simulink model "Simulator_3D"  (R2018a)
settings: Solver=ode4  StartTime=0.0  StopTime=80  FixedStep=T  RelTol=1e-3
values from neighbouring files (symbols this model uses):
  A_w = 1*1.5/2    (= 0.75)    [init_Simulator.m]
  A_w2 = 1*0.27/2    (= 0.135)    [init_Simulator.m]
  epsilon_w = 0    [init_Simulator.m]
  epsilon_w2 = pi    (= 3.14159265359)    [init_Simulator.m]
  k_w = omega_w^2/g    (= 0.123862835563)    [init_Simulator.m]
  k_w2 = omega_w2^2/g    (= 0.447144836384)    [init_Simulator.m]
  Lc_0 = 7    [init_Simulator.m]
  omega_w = 2*pi/T_w    (= 1.10231321179)    [init_Simulator.m]
  omega_w2 = 2*pi/T_w2    (= 2.09439510239)    [init_Simulator.m]
  T = 1/30    (= 0.0333333333333)    [init_Simulator.m]
  w_dir = 1    [init_Simulator.m]
  w_dir2 = 1    [init_Simulator.m]
  zu_bar = X0_b(2) + Lc_0*sin(alpha_bar_0)    [init_Simulator.m]
libraries: vrlib x132
(part 2 of 6)

== system Simulator_3D/Subsystem/5 static wave points6 ==
  t : Inport
  x : Inport  Port=2
  Bias{23,25,27,29,31} (5 alike) : Bias  Bias=10
  Bias{24,26,28,30,32} (5 alike) : Bias  Bias=1
  Display : Display
  Divide : Product  Inputs=*/
  Mux{11..15} (5 alike) : Mux  Inputs=2
  Product : Product
  Round : Rounding
  Subsystem12 : Subsystem
  Subsystem13 : Subsystem
  Subsystem14 : Subsystem
  Subsystem15 : Subsystem
  Subsystem16 : Subsystem
  Sum{,1..4} (5 alike) : Sum  Inputs=|++
  Viewpoint {12..16} (5 alike) : vrlib/VR Signal Expander  outwidth=3  outidx=[1 2]
      settings: SourceProductName=Simulink 3D Animation  SourceProductBaseCode=VR
  reference : Constant  Value=5+3
  window width : Constant  Value=10
  Out1 : Outport
  Out2 : Outport  Port=2
  Out3 : Outport  Port=3
  Out4 : Outport  Port=4
  Out5 : Outport  Port=5
  Out6 : Outport  Port=6
  Out7 : Outport  Port=7
  Out8 : Outport  Port=8
  Out9 : Outport  Port=9
  Out10 : Outport  Port=10
  wires:
  Sum2/1 -> Subsystem15/2(x), Mux14/1
  Sum1/1 -> Subsystem13/2(x), Mux12/1
  Sum3/1 -> Subsystem14/2(x), Mux13/1
  Subsystem14/2(theta) -> Out6/1
  Subsystem13/2(theta) -> Out4/1
  Bias27/1 -> Mux13/2
  Mux13/1 -> Viewpoint 14/1
  Subsystem13/1(zeta) -> Bias25/1
  Subsystem16/2(theta) -> Out10/1
  Mux12/1 -> Viewpoint 13/1
  Bias23/1 -> Mux11/2
  Mux11/1 -> Viewpoint 12/1
  Subsystem14/1(zeta) -> Bias27/1
  Bias25/1 -> Mux12/2
  Subsystem15/2(theta) -> Out8/1
  Mux15/1 -> Viewpoint 16/1
  Bias31/1 -> Mux15/2
  Viewpoint 16/1 -> Out9/1
  Sum4/1 -> Subsystem16/2(x), Mux15/1
  Subsystem12/2(theta) -> Out2/1
  Subsystem16/1(zeta) -> Bias31/1
  Bias29/1 -> Mux14/2
  Sum/1 -> Subsystem12/2(x), Mux11/1
  Mux14/1 -> Viewpoint 15/1
  Viewpoint 12/1 -> Display/1, Out1/1
  Subsystem12/1(zeta) -> Bias23/1
  Viewpoint 15/1 -> Out7/1
  Subsystem15/1(zeta) -> Bias29/1
  t/1 -> Subsystem15/1(t), Subsystem16/1(t), Subsystem14/1(t), Subsystem13/1(t), Subsystem12/1(t)
  Round/1 -> Product/2
  Divide/1 -> Round/1
  x/1 -> Divide/1
  window width/1 -> Divide/2, Product/1
  Bias24/1 -> Bias26/1, Sum/1
  reference/1 -> Bias24/1
  Product/1 -> Sum4/2, Sum2/2, Sum3/2, Sum1/2, Sum/2
  Bias26/1 -> Bias28/1, Sum1/1
  Bias32/1 -> Sum4/1
  Bias30/1 -> Bias32/1, Sum2/1
  Bias28/1 -> Bias30/1, Sum3/1
  Viewpoint 13/1 -> Out3/1
  Viewpoint 14/1 -> Out5/1

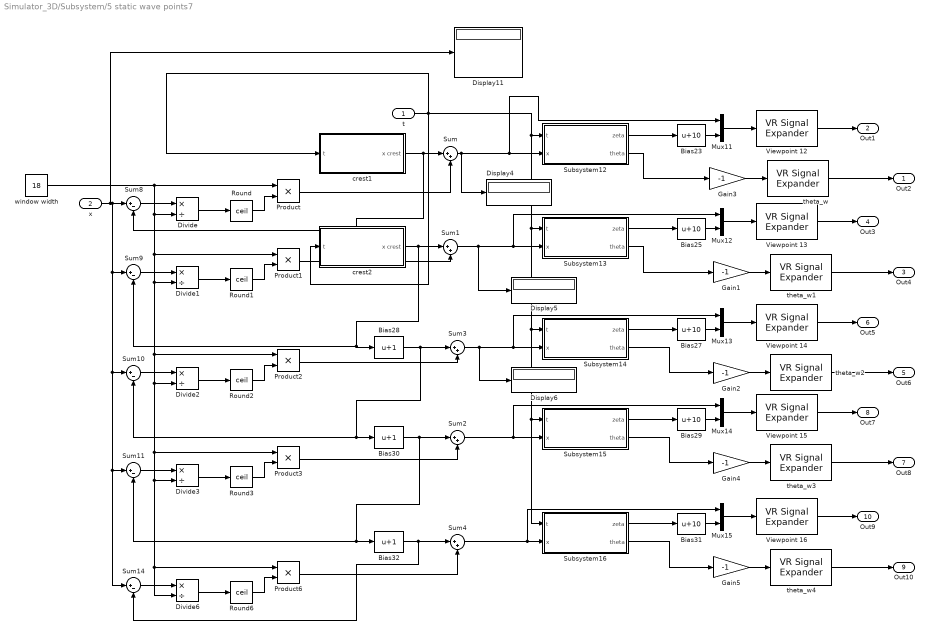
== system Simulator_3D/Subsystem/5 static wave points7 ==
  t : Inport
  x : Inport  Port=2
  Bias{23,25,27,29,31} (5 alike) : Bias  Bias=10
  Bias28 : Bias  Bias=1
  Bias30 : Bias  Bias=1
  Bias32 : Bias  Bias=1
  Display{4..6,11} (4 alike) : Display
  Divide{,1..3,6} (5 alike) : Product  Inputs=*/
  Gain{1..5} (5 alike) : Gain  Gain=-1
  Mux{11..15} (5 alike) : Mux  Inputs=2
  Product{,1..3,6} (5 alike) : Product
  Round{,1..3,6} (5 alike) : Rounding  Operator=ceil
  Subsystem12 : Subsystem
  Subsystem13 : Subsystem
  Subsystem14 : Subsystem
  Subsystem15 : Subsystem
  Subsystem16 : Subsystem
  Sum{,1..4} (5 alike) : Sum  Inputs=|++
  Sum{8..11,14} (5 alike) : Sum  Inputs=|+-
  Viewpoint {12..16} (5 alike) : vrlib/VR Signal Expander  outwidth=3  outidx=[1 2]
      settings: SourceProductName=Simulink 3D Animation  SourceProductBaseCode=VR
  crest1 : Subsystem
  crest2 : Subsystem
  theta_w{,1..4} (5 alike) : vrlib/VR Signal Expander  outwidth=4  outidx=[4]
      settings: SourceProductName=Simulink 3D Animation  SourceProductBaseCode=VR
  window width : Constant  Value=18
  Out2 : Outport
  Out1 : Outport  Port=2
  Out4 : Outport  Port=3
  Out3 : Outport  Port=4
  Out6 : Outport  Port=5
  Out5 : Outport  Port=6
  Out8 : Outport  Port=7
  Out7 : Outport  Port=8
  Out10 : Outport  Port=9
  Out9 : Outport  Port=10
  wires:
  x/1 -> Sum8/1, Sum9/1, Sum10/1, Sum11/1, Sum14/1, Display11/1
  window width/1 -> Product/1, Divide/2, Product1/1, Divide1/2, Divide2/2, Divide3/2, Product6/1, Divide6/2, Product3/1, Product2/1
  Round6/1 -> Product6/2
  Divide6/1 -> Round6/1
  Sum14/1 -> Divide6/1
  Product6/1 -> Sum4/2
  Bias32/1 -> Sum4/1, Sum14/2
  Product3/1 -> Sum2/2
  Sum11/1 -> Divide3/1
  Divide3/1 -> Round3/1
  Round3/1 -> Product3/2
  Bias30/1 -> Bias32/1, Sum11/2, Sum2/1
  Bias28/1 -> Sum3/1, Sum10/2, Bias30/1
  Round2/1 -> Product2/2
  Divide2/1 -> Round2/1
  Sum10/1 -> Divide2/1
  Product2/1 -> Sum3/2
  Product1/1 -> Sum1/2
  Sum9/1 -> Divide1/1
  Divide1/1 -> Round1/1
  Round1/1 -> Product1/2
  crest2/1(x crest) -> Bias28/1, Sum9/2, Sum1/1
  crest1/1(x crest) -> Sum/1, Sum8/2
  t/1 -> crest2/1(t), crest1/1(t), Subsystem15/1(t), Subsystem16/1(t), Subsystem14/1(t), Subsystem13/1(t), Subsystem12/1(t)
  Round/1 -> Product/2
  Divide/1 -> Round/1
  Sum8/1 -> Divide/1
  Subsystem13/2(theta) -> Gain1/1
  Gain2/1 -> theta_w2/1
  Gain4/1 -> theta_w3/1
  theta_w1/1 -> Out4/1
  Subsystem16/2(theta) -> Gain5/1
  Viewpoint 15/1 -> Out7/1
  Sum2/1 -> Subsystem15/2(x), Mux14/1
  Sum1/1 -> Subsystem13/2(x), Mux12/1, Display5/1
  Sum4/1 -> Mux15/1, Subsystem16/2(x)
  Subsystem15/2(theta) -> Gain4/1
  Bias27/1 -> Mux13/2
  Bias25/1 -> Mux12/2
  Mux13/1 -> Viewpoint 14/1
  Subsystem13/1(zeta) -> Bias25/1
  Viewpoint 14/1 -> Out5/1
  Viewpoint 16/1 -> Out9/1
  Bias23/1 -> Mux11/2
  Mux15/1 -> Viewpoint 16/1
  Subsystem14/1(zeta) -> Bias27/1
  Bias31/1 -> Mux15/2
  Subsystem14/2(theta) -> Gain2/1
  Mux14/1 -> Viewpoint 15/1
  Subsystem16/1(zeta) -> Bias31/1
  Subsystem15/1(zeta) -> Bias29/1
  Sum/1 -> Mux11/1, Subsystem12/2(x), Display4/1
  Viewpoint 13/1 -> Out3/1
  Subsystem12/1(zeta) -> Bias23/1
  Gain5/1 -> theta_w4/1
  theta_w3/1 -> Out8/1
  Mux11/1 -> Viewpoint 12/1
  Subsystem12/2(theta) -> Gain3/1
  Bias29/1 -> Mux14/2
  theta_w2/1 -> Out6/1
  Gain1/1 -> theta_w1/1
  Viewpoint 12/1 -> Out1/1
  theta_w4/1 -> Out10/1
  Sum3/1 -> Subsystem14/2(x), Mux13/1, Display6/1
  theta_w/1 -> Out2/1
  Mux12/1 -> Viewpoint 13/1
  Gain3/1 -> theta_w/1
  Product/1 -> Sum/2

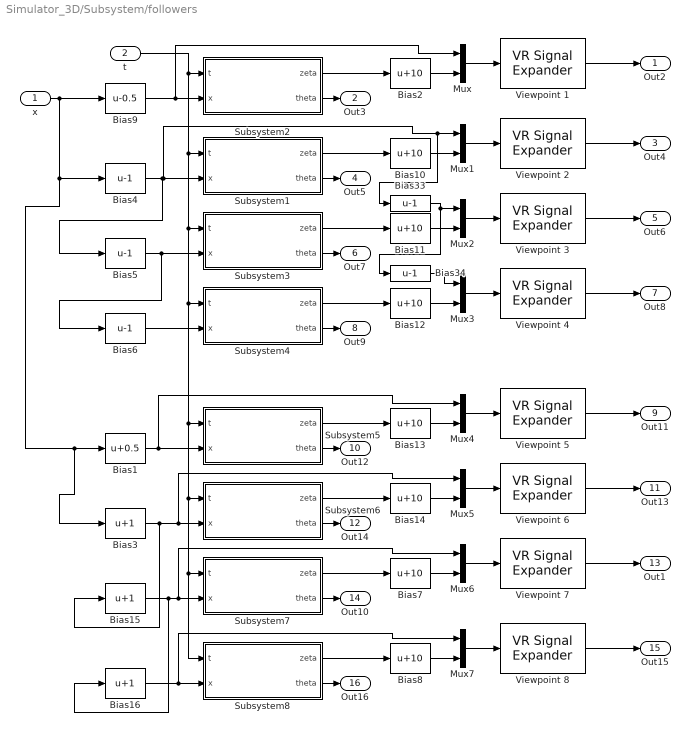
== system Simulator_3D/Subsystem/followers ==
  x : Inport
  t : Inport  Port=2
  Bias1 : Bias  Bias=0.5
  Bias{2,7..8,10..14} (8 alike) : Bias  Bias=10
  Bias15 : Bias  Bias=1
  Bias16 : Bias  Bias=1
  Bias3 : Bias  Bias=1
  Bias{4..6,33..34} (5 alike) : Bias  Bias=-1
  Bias9 : Bias  Bias=-0.5
  Mux{,1..7} (8 alike) : Mux  Inputs=2
  Subsystem1 : Subsystem
  Subsystem2 : Subsystem
  Subsystem3 : Subsystem
  Subsystem4 : Subsystem
  Subsystem5 : Subsystem
  Subsystem6 : Subsystem
  Subsystem7 : Subsystem
  Subsystem8 : Subsystem
  Viewpoint {1..8} (8 alike) : vrlib/VR Signal Expander  outwidth=3  outidx=[1 2]
      settings: SourceProductName=Simulink 3D Animation  SourceProductBaseCode=VR
  Out2 : Outport
  Out3 : Outport  Port=2
  Out4 : Outport  Port=3
  Out5 : Outport  Port=4
  Out6 : Outport  Port=5
  Out7 : Outport  Port=6
  Out8 : Outport  Port=7
  Out9 : Outport  Port=8
  Out11 : Outport  Port=9
  Out12 : Outport  Port=10
  Out13 : Outport  Port=11
  Out14 : Outport  Port=12
  Out1 : Outport  Port=13
  Out10 : Outport  Port=14
  Out15 : Outport  Port=15
  Out16 : Outport  Port=16
  wires:
  Subsystem2/2(theta) -> Out3/1
  Bias33/1 -> Bias34/1, Mux2/1
  Subsystem6/2(theta) -> Out14/1
  Mux2/1 -> Viewpoint 3/1
  Bias4/1 -> Bias5/1, Bias33/1, Mux1/1, Subsystem1/2(x)
  Mux5/1 -> Viewpoint 6/1
  Bias11/1 -> Mux2/2
  Mux/1 -> Viewpoint 1/1
  Bias13/1 -> Mux4/2
  Subsystem2/1(zeta) -> Bias2/1
  Subsystem3/1(zeta) -> Bias11/1
  Bias10/1 -> Mux1/2
  Bias34/1 -> Mux3/1
  Mux4/1 -> Viewpoint 5/1
  Bias2/1 -> Mux/2
  Mux3/1 -> Viewpoint 4/1
  Bias14/1 -> Mux5/2
  Viewpoint 4/1 -> Out8/1
  Bias5/1 -> Bias6/1, Subsystem3/2(x)
  Viewpoint 6/1 -> Out13/1
  Subsystem6/1(zeta) -> Bias14/1
  Subsystem4/1(zeta) -> Bias12/1
  Subsystem3/2(theta) -> Out7/1
  Subsystem1/1(zeta) -> Bias10/1
  Subsystem5/1(zeta) -> Bias13/1
  Bias9/1 -> Mux/1, Subsystem2/2(x)
  Viewpoint 1/1 -> Out2/1
  Bias6/1 -> Subsystem4/2(x)
  Viewpoint 2/1 -> Out4/1
  Bias12/1 -> Mux3/2
  Mux1/1 -> Viewpoint 2/1
  Subsystem4/2(theta) -> Out9/1
  Viewpoint 3/1 -> Out6/1
  Viewpoint 5/1 -> Out11/1
  Subsystem1/2(theta) -> Out5/1
  Subsystem5/2(theta) -> Out12/1
  x/1 -> Bias3/1, Bias1/1, Bias4/1, Bias9/1
  Bias1/1 -> Mux4/1, Subsystem5/2(x)
  Subsystem7/1(zeta) -> Bias7/1
  Viewpoint 7/1 -> Out1/1
  Bias7/1 -> Mux6/2
  Mux6/1 -> Viewpoint 7/1
  Bias15/1 -> Subsystem7/2(x), Mux6/1, Bias16/1
  Subsystem7/2(theta) -> Out10/1
  Subsystem8/2(theta) -> Out16/1
  Bias3/1 -> Bias15/1, Mux5/1, Subsystem6/2(x)
  Bias16/1 -> Mux7/1, Subsystem8/2(x)
  Mux7/1 -> Viewpoint 8/1
  Bias8/1 -> Mux7/2
  Viewpoint 8/1 -> Out15/1
  Subsystem8/1(zeta) -> Bias8/1
  t/1 -> Subsystem1/1(t), Subsystem3/1(t), Subsystem4/1(t), Subsystem5/1(t), Subsystem8/1(t), Subsystem7/1(t), Subsystem6/1(t), Subsystem2/1(t)

== system Simulator_3D/Subsystem1/Subsystem1 ==
  t : Inport
  x : Inport  Port=2
  Subsystem : Subsystem
  Subsystem1 : Subsystem
  Sum2 : Sum  Inputs=++|
  zeta : Outport
  wires:
  Subsystem1/1(zeta(x,t)) -> Sum2/1
  Sum2/1 -> zeta/1
  Subsystem/1(zeta(x,t)) -> Sum2/2
  t/1 -> Subsystem1/1(t), Subsystem/1(t)
  x/1 -> Subsystem1/2(x), Subsystem/2(x)

== system Simulator_3D/Subsystem1/Subsystem10 ==
  t : Inport
  x : Inport  Port=2
  Subsystem : Subsystem
  Subsystem1 : Subsystem
  Sum2 : Sum  Inputs=++|
  zeta : Outport
  wires:
  x/1 -> Subsystem/2(x), Subsystem1/2(x)
  t/1 -> Subsystem/1(t), Subsystem1/1(t)
  Subsystem/1(zeta(x,t)) -> Sum2/2
  Sum2/1 -> zeta/1
  Subsystem1/1(zeta(x,t)) -> Sum2/1

== system Simulator_3D/Subsystem1/Subsystem11 ==
  t : Inport
  x : Inport  Port=2
  Subsystem : Subsystem
  Subsystem1 : Subsystem
  Sum2 : Sum  Inputs=++|
  zeta : Outport
  wires:
  Subsystem1/1(zeta(x,t)) -> Sum2/1
  Sum2/1 -> zeta/1
  Subsystem/1(zeta(x,t)) -> Sum2/2
  t/1 -> Subsystem1/1(t), Subsystem/1(t)
  x/1 -> Subsystem1/2(x), Subsystem/2(x)

== system Simulator_3D/Subsystem1/Subsystem12 ==
  t : Inport
  x : Inport  Port=2
  Subsystem : Subsystem
  Subsystem1 : Subsystem
  Sum2 : Sum  Inputs=++|
  zeta : Outport
  wires:
  x/1 -> Subsystem/2(x), Subsystem1/2(x)
  t/1 -> Subsystem/1(t), Subsystem1/1(t)
  Subsystem/1(zeta(x,t)) -> Sum2/2
  Sum2/1 -> zeta/1
  Subsystem1/1(zeta(x,t)) -> Sum2/1

== system Simulator_3D/Subsystem1/Subsystem13 ==
  t : Inport
  x : Inport  Port=2
  Subsystem : Subsystem
  Subsystem1 : Subsystem
  Sum2 : Sum  Inputs=++|
  zeta : Outport
  wires:
  Subsystem1/1(zeta(x,t)) -> Sum2/1
  Sum2/1 -> zeta/1
  Subsystem/1(zeta(x,t)) -> Sum2/2
  t/1 -> Subsystem1/1(t), Subsystem/1(t)
  x/1 -> Subsystem1/2(x), Subsystem/2(x)

== system Simulator_3D/Subsystem1/Subsystem14 ==
  t : Inport
  x : Inport  Port=2
  Subsystem : Subsystem
  Subsystem1 : Subsystem
  Sum2 : Sum  Inputs=++|
  zeta : Outport
  wires:
  x/1 -> Subsystem/2(x), Subsystem1/2(x)
  t/1 -> Subsystem/1(t), Subsystem1/1(t)
  Subsystem/1(zeta(x,t)) -> Sum2/2
  Sum2/1 -> zeta/1
  Subsystem1/1(zeta(x,t)) -> Sum2/1

== system Simulator_3D/Subsystem1/Subsystem15 ==
  t : Inport
  x : Inport  Port=2
  Subsystem : Subsystem
  Subsystem1 : Subsystem
  Sum2 : Sum  Inputs=++|
  zeta : Outport
  wires:
  Subsystem1/1(zeta(x,t)) -> Sum2/1
  Sum2/1 -> zeta/1
  Subsystem/1(zeta(x,t)) -> Sum2/2
  t/1 -> Subsystem1/1(t), Subsystem/1(t)
  x/1 -> Subsystem1/2(x), Subsystem/2(x)

== system Simulator_3D/Subsystem1/Subsystem16 ==
  t : Inport
  x : Inport  Port=2
  Subsystem : Subsystem
  Subsystem1 : Subsystem
  Sum2 : Sum  Inputs=++|
  zeta : Outport
  wires:
  x/1 -> Subsystem/2(x), Subsystem1/2(x)
  t/1 -> Subsystem/1(t), Subsystem1/1(t)
  Subsystem/1(zeta(x,t)) -> Sum2/2
  Sum2/1 -> zeta/1
  Subsystem1/1(zeta(x,t)) -> Sum2/1

== system Simulator_3D/Subsystem1/Subsystem2 ==
  t : Inport
  x : Inport  Port=2
  Subsystem : Subsystem
  Subsystem1 : Subsystem
  Sum2 : Sum  Inputs=++|
  zeta : Outport
  wires:
  x/1 -> Subsystem/2(x), Subsystem1/2(x)
  t/1 -> Subsystem/1(t), Subsystem1/1(t)
  Subsystem/1(zeta(x,t)) -> Sum2/2
  Sum2/1 -> zeta/1
  Subsystem1/1(zeta(x,t)) -> Sum2/1

== system Simulator_3D/Subsystem1/Subsystem3 ==
  t : Inport
  x : Inport  Port=2
  Subsystem : Subsystem
  Subsystem1 : Subsystem
  Sum2 : Sum  Inputs=++|
  zeta : Outport
  wires:
  Subsystem1/1(zeta(x,t)) -> Sum2/1
  Sum2/1 -> zeta/1
  Subsystem/1(zeta(x,t)) -> Sum2/2
  t/1 -> Subsystem1/1(t), Subsystem/1(t)
  x/1 -> Subsystem1/2(x), Subsystem/2(x)

== system Simulator_3D/Subsystem1/Subsystem4 ==
  t : Inport
  x : Inport  Port=2
  Subsystem : Subsystem
  Subsystem1 : Subsystem
  Sum2 : Sum  Inputs=++|
  zeta : Outport
  wires:
  x/1 -> Subsystem/2(x), Subsystem1/2(x)
  t/1 -> Subsystem/1(t), Subsystem1/1(t)
  Subsystem/1(zeta(x,t)) -> Sum2/2
  Sum2/1 -> zeta/1
  Subsystem1/1(zeta(x,t)) -> Sum2/1

== system Simulator_3D/Subsystem1/Subsystem5 ==
  t : Inport
  x : Inport  Port=2
  Subsystem : Subsystem
  Subsystem1 : Subsystem
  Sum2 : Sum  Inputs=++|
  zeta : Outport
  wires:
  Subsystem1/1(zeta(x,t)) -> Sum2/1
  Sum2/1 -> zeta/1
  Subsystem/1(zeta(x,t)) -> Sum2/2
  t/1 -> Subsystem1/1(t), Subsystem/1(t)
  x/1 -> Subsystem1/2(x), Subsystem/2(x)

== system Simulator_3D/Subsystem1/Subsystem6 ==
  t : Inport
  x : Inport  Port=2
  Subsystem : Subsystem
  Subsystem1 : Subsystem
  Sum2 : Sum  Inputs=++|
  zeta : Outport
  wires:
  x/1 -> Subsystem/2(x), Subsystem1/2(x)
  t/1 -> Subsystem/1(t), Subsystem1/1(t)
  Subsystem/1(zeta(x,t)) -> Sum2/2
  Sum2/1 -> zeta/1
  Subsystem1/1(zeta(x,t)) -> Sum2/1

== system Simulator_3D/Subsystem1/Subsystem7 ==
  t : Inport
  x : Inport  Port=2
  Subsystem : Subsystem
  Subsystem1 : Subsystem
  Sum2 : Sum  Inputs=++|
  zeta : Outport
  wires:
  Subsystem1/1(zeta(x,t)) -> Sum2/1
  Sum2/1 -> zeta/1
  Subsystem/1(zeta(x,t)) -> Sum2/2
  t/1 -> Subsystem1/1(t), Subsystem/1(t)
  x/1 -> Subsystem1/2(x), Subsystem/2(x)

== system Simulator_3D/Subsystem1/Subsystem8 ==
  t : Inport
  x : Inport  Port=2
  Subsystem : Subsystem
  Subsystem1 : Subsystem
  Sum2 : Sum  Inputs=++|
  zeta : Outport
  wires:
  x/1 -> Subsystem/2(x), Subsystem1/2(x)
  t/1 -> Subsystem/1(t), Subsystem1/1(t)
  Subsystem/1(zeta(x,t)) -> Sum2/2
  Sum2/1 -> zeta/1
  Subsystem1/1(zeta(x,t)) -> Sum2/1

== system Simulator_3D/Subsystem1/Subsystem9 ==
  t : Inport
  x : Inport  Port=2
  Subsystem : Subsystem
  Subsystem1 : Subsystem
  Sum2 : Sum  Inputs=++|
  zeta : Outport
  wires:
  Subsystem1/1(zeta(x,t)) -> Sum2/1
  Sum2/1 -> zeta/1
  Subsystem/1(zeta(x,t)) -> Sum2/2
  t/1 -> Subsystem1/1(t), Subsystem/1(t)
  x/1 -> Subsystem1/2(x), Subsystem/2(x)

== system Simulator_3D/Subsystem2/Subsystem1 ==
  t : Inport
  x : Inport  Port=2
  Subsystem : Subsystem
  Subsystem1 : Subsystem
  Sum1 : Sum  Inputs=++|
  Sum2 : Sum  Inputs=++|
  zeta : Outport
  theta : Outport  Port=2
  wires:
  Sum1/1 -> theta/1
  Subsystem1/2(theta) -> Sum1/1
  Subsystem/2(theta) -> Sum1/2
  Subsystem1/1(zeta(x,t)) -> Sum2/1
  Sum2/1 -> zeta/1
  Subsystem/1(zeta(x,t)) -> Sum2/2
  t/1 -> Subsystem1/1(t), Subsystem/1(t)
  x/1 -> Subsystem1/2(x), Subsystem/2(x)

== system Simulator_3D/Subsystem2/Subsystem10 ==
  t : Inport
  x : Inport  Port=2
  Subsystem : Subsystem
  Subsystem1 : Subsystem
  Sum1 : Sum  Inputs=++|
  Sum2 : Sum  Inputs=++|
  zeta : Outport
  theta : Outport  Port=2
  wires:
  Sum1/1 -> theta/1
  Subsystem1/2(theta) -> Sum1/1
  Subsystem/2(theta) -> Sum1/2
  Subsystem1/1(zeta(x,t)) -> Sum2/1
  Sum2/1 -> zeta/1
  Subsystem/1(zeta(x,t)) -> Sum2/2
  t/1 -> Subsystem1/1(t), Subsystem/1(t)
  x/1 -> Subsystem1/2(x), Subsystem/2(x)

== system Simulator_3D/Subsystem2/Subsystem11 ==
  t : Inport
  x : Inport  Port=2
  Subsystem : Subsystem
  Subsystem1 : Subsystem
  Sum1 : Sum  Inputs=++|
  Sum2 : Sum  Inputs=++|
  zeta : Outport
  theta : Outport  Port=2
  wires:
  x/1 -> Subsystem/2(x), Subsystem1/2(x)
  t/1 -> Subsystem/1(t), Subsystem1/1(t)
  Subsystem/1(zeta(x,t)) -> Sum2/2
  Sum2/1 -> zeta/1
  Subsystem1/1(zeta(x,t)) -> Sum2/1
  Subsystem/2(theta) -> Sum1/2
  Subsystem1/2(theta) -> Sum1/1
  Sum1/1 -> theta/1

== system Simulator_3D/Subsystem2/Subsystem12 ==
  t : Inport
  x : Inport  Port=2
  Subsystem : Subsystem
  Subsystem1 : Subsystem
  Sum1 : Sum  Inputs=++|
  Sum2 : Sum  Inputs=++|
  zeta : Outport
  theta : Outport  Port=2
  wires:
  Sum1/1 -> theta/1
  Subsystem1/2(theta) -> Sum1/1
  Subsystem/2(theta) -> Sum1/2
  Subsystem1/1(zeta(x,t)) -> Sum2/1
  Sum2/1 -> zeta/1
  Subsystem/1(zeta(x,t)) -> Sum2/2
  t/1 -> Subsystem1/1(t), Subsystem/1(t)
  x/1 -> Subsystem1/2(x), Subsystem/2(x)

== system Simulator_3D/Subsystem2/Subsystem13 ==
  t : Inport
  x : Inport  Port=2
  Subsystem : Subsystem
  Subsystem1 : Subsystem
  Sum1 : Sum  Inputs=++|
  Sum2 : Sum  Inputs=++|
  zeta : Outport
  theta : Outport  Port=2
  wires:
  x/1 -> Subsystem/2(x), Subsystem1/2(x)
  t/1 -> Subsystem/1(t), Subsystem1/1(t)
  Subsystem/1(zeta(x,t)) -> Sum2/2
  Sum2/1 -> zeta/1
  Subsystem1/1(zeta(x,t)) -> Sum2/1
  Subsystem/2(theta) -> Sum1/2
  Subsystem1/2(theta) -> Sum1/1
  Sum1/1 -> theta/1

== system Simulator_3D/Subsystem2/Subsystem14 ==
  t : Inport
  x : Inport  Port=2
  Subsystem : Subsystem
  Subsystem1 : Subsystem
  Sum1 : Sum  Inputs=++|
  Sum2 : Sum  Inputs=++|
  zeta : Outport
  theta : Outport  Port=2
  wires:
  Sum1/1 -> theta/1
  Subsystem1/2(theta) -> Sum1/1
  Subsystem/2(theta) -> Sum1/2
  Subsystem1/1(zeta(x,t)) -> Sum2/1
  Sum2/1 -> zeta/1
  Subsystem/1(zeta(x,t)) -> Sum2/2
  t/1 -> Subsystem1/1(t), Subsystem/1(t)
  x/1 -> Subsystem1/2(x), Subsystem/2(x)

== system Simulator_3D/Subsystem2/Subsystem15 ==
  t : Inport
  x : Inport  Port=2
  Subsystem : Subsystem
  Subsystem1 : Subsystem
  Sum1 : Sum  Inputs=++|
  Sum2 : Sum  Inputs=++|
  zeta : Outport
  theta : Outport  Port=2
  wires:
  x/1 -> Subsystem/2(x), Subsystem1/2(x)
  t/1 -> Subsystem/1(t), Subsystem1/1(t)
  Subsystem/1(zeta(x,t)) -> Sum2/2
  Sum2/1 -> zeta/1
  Subsystem1/1(zeta(x,t)) -> Sum2/1
  Subsystem/2(theta) -> Sum1/2
  Subsystem1/2(theta) -> Sum1/1
  Sum1/1 -> theta/1

== system Simulator_3D/Subsystem2/Subsystem16 ==
  t : Inport
  x : Inport  Port=2
  Subsystem : Subsystem
  Subsystem1 : Subsystem
  Sum1 : Sum  Inputs=++|
  Sum2 : Sum  Inputs=++|
  zeta : Outport
  theta : Outport  Port=2
  wires:
  Sum1/1 -> theta/1
  Subsystem1/2(theta) -> Sum1/1
  Subsystem/2(theta) -> Sum1/2
  Subsystem1/1(zeta(x,t)) -> Sum2/1
  Sum2/1 -> zeta/1
  Subsystem/1(zeta(x,t)) -> Sum2/2
  t/1 -> Subsystem1/1(t), Subsystem/1(t)
  x/1 -> Subsystem1/2(x), Subsystem/2(x)

== system Simulator_3D/Subsystem2/Subsystem2 ==
  t : Inport
  x : Inport  Port=2
  Subsystem : Subsystem
  Subsystem1 : Subsystem
  Sum1 : Sum  Inputs=++|
  Sum2 : Sum  Inputs=++|
  zeta : Outport
  theta : Outport  Port=2
  wires:
  x/1 -> Subsystem/2(x), Subsystem1/2(x)
  t/1 -> Subsystem/1(t), Subsystem1/1(t)
  Subsystem/1(zeta(x,t)) -> Sum2/2
  Sum2/1 -> zeta/1
  Subsystem1/1(zeta(x,t)) -> Sum2/1
  Subsystem/2(theta) -> Sum1/2
  Subsystem1/2(theta) -> Sum1/1
  Sum1/1 -> theta/1

== system Simulator_3D/Subsystem2/Subsystem3 ==
  t : Inport
  x : Inport  Port=2
  Subsystem : Subsystem
  Subsystem1 : Subsystem
  Sum1 : Sum  Inputs=++|
  Sum2 : Sum  Inputs=++|
  zeta : Outport
  theta : Outport  Port=2
  wires:
  x/1 -> Subsystem/2(x), Subsystem1/2(x)
  t/1 -> Subsystem/1(t), Subsystem1/1(t)
  Subsystem/1(zeta(x,t)) -> Sum2/2
  Sum2/1 -> zeta/1
  Subsystem1/1(zeta(x,t)) -> Sum2/1
  Subsystem/2(theta) -> Sum1/2
  Subsystem1/2(theta) -> Sum1/1
  Sum1/1 -> theta/1

== system Simulator_3D/Subsystem2/Subsystem4 ==
  t : Inport
  x : Inport  Port=2
  Subsystem : Subsystem
  Subsystem1 : Subsystem
  Sum1 : Sum  Inputs=++|
  Sum2 : Sum  Inputs=++|
  zeta : Outport
  theta : Outport  Port=2
  wires:
  Sum1/1 -> theta/1
  Subsystem1/2(theta) -> Sum1/1
  Subsystem/2(theta) -> Sum1/2
  Subsystem1/1(zeta(x,t)) -> Sum2/1
  Sum2/1 -> zeta/1
  Subsystem/1(zeta(x,t)) -> Sum2/2
  t/1 -> Subsystem1/1(t), Subsystem/1(t)
  x/1 -> Subsystem1/2(x), Subsystem/2(x)

== system Simulator_3D/Subsystem2/Subsystem5 ==
  t : Inport
  x : Inport  Port=2
  Subsystem : Subsystem
  Subsystem1 : Subsystem
  Sum1 : Sum  Inputs=++|
  Sum2 : Sum  Inputs=++|
  zeta : Outport
  theta : Outport  Port=2
  wires:
  x/1 -> Subsystem/2(x), Subsystem1/2(x)
  t/1 -> Subsystem/1(t), Subsystem1/1(t)
  Subsystem/1(zeta(x,t)) -> Sum2/2
  Sum2/1 -> zeta/1
  Subsystem1/1(zeta(x,t)) -> Sum2/1
  Subsystem/2(theta) -> Sum1/2
  Subsystem1/2(theta) -> Sum1/1
  Sum1/1 -> theta/1

== system Simulator_3D/Subsystem2/Subsystem6 ==
  t : Inport
  x : Inport  Port=2
  Subsystem : Subsystem
  Subsystem1 : Subsystem
  Sum1 : Sum  Inputs=++|
  Sum2 : Sum  Inputs=++|
  zeta : Outport
  theta : Outport  Port=2
  wires:
  Sum1/1 -> theta/1
  Subsystem1/2(theta) -> Sum1/1
  Subsystem/2(theta) -> Sum1/2
  Subsystem1/1(zeta(x,t)) -> Sum2/1
  Sum2/1 -> zeta/1
  Subsystem/1(zeta(x,t)) -> Sum2/2
  t/1 -> Subsystem1/1(t), Subsystem/1(t)
  x/1 -> Subsystem1/2(x), Subsystem/2(x)

== system Simulator_3D/Subsystem2/Subsystem7 ==
  t : Inport
  x : Inport  Port=2
  Subsystem : Subsystem
  Subsystem1 : Subsystem
  Sum1 : Sum  Inputs=++|
  Sum2 : Sum  Inputs=++|
  zeta : Outport
  theta : Outport  Port=2
  wires:
  x/1 -> Subsystem/2(x), Subsystem1/2(x)
  t/1 -> Subsystem/1(t), Subsystem1/1(t)
  Subsystem/1(zeta(x,t)) -> Sum2/2
  Sum2/1 -> zeta/1
  Subsystem1/1(zeta(x,t)) -> Sum2/1
  Subsystem/2(theta) -> Sum1/2
  Subsystem1/2(theta) -> Sum1/1
  Sum1/1 -> theta/1

== system Simulator_3D/Subsystem2/Subsystem8 ==
  t : Inport
  x : Inport  Port=2
  Subsystem : Subsystem
  Subsystem1 : Subsystem
  Sum1 : Sum  Inputs=++|
  Sum2 : Sum  Inputs=++|
  zeta : Outport
  theta : Outport  Port=2
  wires:
  Sum1/1 -> theta/1
  Subsystem1/2(theta) -> Sum1/1
  Subsystem/2(theta) -> Sum1/2
  Subsystem1/1(zeta(x,t)) -> Sum2/1
  Sum2/1 -> zeta/1
  Subsystem/1(zeta(x,t)) -> Sum2/2
  t/1 -> Subsystem1/1(t), Subsystem/1(t)
  x/1 -> Subsystem1/2(x), Subsystem/2(x)

== system Simulator_3D/Subsystem2/Subsystem9 ==
  t : Inport
  x : Inport  Port=2
  Subsystem : Subsystem
  Subsystem1 : Subsystem
  Sum1 : Sum  Inputs=++|
  Sum2 : Sum  Inputs=++|
  zeta : Outport
  theta : Outport  Port=2
  wires:
  x/1 -> Subsystem/2(x), Subsystem1/2(x)
  t/1 -> Subsystem/1(t), Subsystem1/1(t)
  Subsystem/1(zeta(x,t)) -> Sum2/2
  Sum2/1 -> zeta/1
  Subsystem1/1(zeta(x,t)) -> Sum2/1
  Subsystem/2(theta) -> Sum1/2
  Subsystem1/2(theta) -> Sum1/1
  Sum1/1 -> theta/1

== system Simulator_3D/Subsystem3/Subsystem1 ==
  t : Inport
  x : Inport  Port=2
  Subsystem : Subsystem
  Subsystem1 : Subsystem
  Sum1 : Sum  Inputs=++|
  Sum2 : Sum  Inputs=++|
  zeta : Outport
  theta : Outport  Port=2
  wires:
  Sum1/1 -> theta/1
  Subsystem1/2(theta) -> Sum1/1
  Subsystem/2(theta) -> Sum1/2
  Subsystem1/1(zeta(x,t)) -> Sum2/1
  Sum2/1 -> zeta/1
  Subsystem/1(zeta(x,t)) -> Sum2/2
  t/1 -> Subsystem1/1(t), Subsystem/1(t)
  x/1 -> Subsystem1/2(x), Subsystem/2(x)

== system Simulator_3D/Subsystem3/Subsystem10 ==
  t : Inport
  x : Inport  Port=2
  Subsystem : Subsystem
  Subsystem1 : Subsystem
  Sum1 : Sum  Inputs=++|
  Sum2 : Sum  Inputs=++|
  zeta : Outport
  theta : Outport  Port=2
  wires:
  Sum1/1 -> theta/1
  Subsystem1/2(theta) -> Sum1/1
  Subsystem/2(theta) -> Sum1/2
  Subsystem1/1(zeta(x,t)) -> Sum2/1
  Sum2/1 -> zeta/1
  Subsystem/1(zeta(x,t)) -> Sum2/2
  t/1 -> Subsystem1/1(t), Subsystem/1(t)
  x/1 -> Subsystem1/2(x), Subsystem/2(x)

== system Simulator_3D/Subsystem3/Subsystem11 ==
  t : Inport
  x : Inport  Port=2
  Subsystem : Subsystem
  Subsystem1 : Subsystem
  Sum1 : Sum  Inputs=++|
  Sum2 : Sum  Inputs=++|
  zeta : Outport
  theta : Outport  Port=2
  wires:
  x/1 -> Subsystem/2(x), Subsystem1/2(x)
  t/1 -> Subsystem/1(t), Subsystem1/1(t)
  Subsystem/1(zeta(x,t)) -> Sum2/2
  Sum2/1 -> zeta/1
  Subsystem1/1(zeta(x,t)) -> Sum2/1
  Subsystem/2(theta) -> Sum1/2
  Subsystem1/2(theta) -> Sum1/1
  Sum1/1 -> theta/1

== system Simulator_3D/Subsystem3/Subsystem12 ==
  t : Inport
  x : Inport  Port=2
  Subsystem : Subsystem
  Subsystem1 : Subsystem
  Sum1 : Sum  Inputs=++|
  Sum2 : Sum  Inputs=++|
  zeta : Outport
  theta : Outport  Port=2
  wires:
  Sum1/1 -> theta/1
  Subsystem1/2(theta) -> Sum1/1
  Subsystem/2(theta) -> Sum1/2
  Subsystem1/1(zeta(x,t)) -> Sum2/1
  Sum2/1 -> zeta/1
  Subsystem/1(zeta(x,t)) -> Sum2/2
  t/1 -> Subsystem1/1(t), Subsystem/1(t)
  x/1 -> Subsystem1/2(x), Subsystem/2(x)

== system Simulator_3D/Subsystem3/Subsystem13 ==
  t : Inport
  x : Inport  Port=2
  Subsystem : Subsystem
  Subsystem1 : Subsystem
  Sum1 : Sum  Inputs=++|
  Sum2 : Sum  Inputs=++|
  zeta : Outport
  theta : Outport  Port=2
  wires:
  x/1 -> Subsystem/2(x), Subsystem1/2(x)
  t/1 -> Subsystem/1(t), Subsystem1/1(t)
  Subsystem/1(zeta(x,t)) -> Sum2/2
  Sum2/1 -> zeta/1
  Subsystem1/1(zeta(x,t)) -> Sum2/1
  Subsystem/2(theta) -> Sum1/2
  Subsystem1/2(theta) -> Sum1/1
  Sum1/1 -> theta/1

== system Simulator_3D/Subsystem3/Subsystem14 ==
  t : Inport
  x : Inport  Port=2
  Subsystem : Subsystem
  Subsystem1 : Subsystem
  Sum1 : Sum  Inputs=++|
  Sum2 : Sum  Inputs=++|
  zeta : Outport
  theta : Outport  Port=2
  wires:
  Sum1/1 -> theta/1
  Subsystem1/2(theta) -> Sum1/1
  Subsystem/2(theta) -> Sum1/2
  Subsystem1/1(zeta(x,t)) -> Sum2/1
  Sum2/1 -> zeta/1
  Subsystem/1(zeta(x,t)) -> Sum2/2
  t/1 -> Subsystem1/1(t), Subsystem/1(t)
  x/1 -> Subsystem1/2(x), Subsystem/2(x)

== system Simulator_3D/Subsystem3/Subsystem15 ==
  t : Inport
  x : Inport  Port=2
  Subsystem : Subsystem
  Subsystem1 : Subsystem
  Sum1 : Sum  Inputs=++|
  Sum2 : Sum  Inputs=++|
  zeta : Outport
  theta : Outport  Port=2
  wires:
  x/1 -> Subsystem/2(x), Subsystem1/2(x)
  t/1 -> Subsystem/1(t), Subsystem1/1(t)
  Subsystem/1(zeta(x,t)) -> Sum2/2
  Sum2/1 -> zeta/1
  Subsystem1/1(zeta(x,t)) -> Sum2/1
  Subsystem/2(theta) -> Sum1/2
  Subsystem1/2(theta) -> Sum1/1
  Sum1/1 -> theta/1

== system Simulator_3D/Subsystem3/Subsystem16 ==
  t : Inport
  x : Inport  Port=2
  Subsystem : Subsystem
  Subsystem1 : Subsystem
  Sum1 : Sum  Inputs=++|
  Sum2 : Sum  Inputs=++|
  zeta : Outport
  theta : Outport  Port=2
  wires:
  Sum1/1 -> theta/1
  Subsystem1/2(theta) -> Sum1/1
  Subsystem/2(theta) -> Sum1/2
  Subsystem1/1(zeta(x,t)) -> Sum2/1
  Sum2/1 -> zeta/1
  Subsystem/1(zeta(x,t)) -> Sum2/2
  t/1 -> Subsystem1/1(t), Subsystem/1(t)
  x/1 -> Subsystem1/2(x), Subsystem/2(x)

== system Simulator_3D/Subsystem3/Subsystem2 ==
  t : Inport
  x : Inport  Port=2
  Subsystem : Subsystem
  Subsystem1 : Subsystem
  Sum1 : Sum  Inputs=++|
  Sum2 : Sum  Inputs=++|
  zeta : Outport
  theta : Outport  Port=2
  wires:
  x/1 -> Subsystem/2(x), Subsystem1/2(x)
  t/1 -> Subsystem/1(t), Subsystem1/1(t)
  Subsystem/1(zeta(x,t)) -> Sum2/2
  Sum2/1 -> zeta/1
  Subsystem1/1(zeta(x,t)) -> Sum2/1
  Subsystem/2(theta) -> Sum1/2
  Subsystem1/2(theta) -> Sum1/1
  Sum1/1 -> theta/1

== system Simulator_3D/Subsystem3/Subsystem3 ==
  t : Inport
  x : Inport  Port=2
  Subsystem : Subsystem
  Subsystem1 : Subsystem
  Sum1 : Sum  Inputs=++|
  Sum2 : Sum  Inputs=++|
  zeta : Outport
  theta : Outport  Port=2
  wires:
  x/1 -> Subsystem/2(x), Subsystem1/2(x)
  t/1 -> Subsystem/1(t), Subsystem1/1(t)
  Subsystem/1(zeta(x,t)) -> Sum2/2
  Sum2/1 -> zeta/1
  Subsystem1/1(zeta(x,t)) -> Sum2/1
  Subsystem/2(theta) -> Sum1/2
  Subsystem1/2(theta) -> Sum1/1
  Sum1/1 -> theta/1

== system Simulator_3D/Subsystem3/Subsystem4 ==
  t : Inport
  x : Inport  Port=2
  Subsystem : Subsystem
  Subsystem1 : Subsystem
  Sum1 : Sum  Inputs=++|
  Sum2 : Sum  Inputs=++|
  zeta : Outport
  theta : Outport  Port=2
  wires:
  Sum1/1 -> theta/1
  Subsystem1/2(theta) -> Sum1/1
  Subsystem/2(theta) -> Sum1/2
  Subsystem1/1(zeta(x,t)) -> Sum2/1
  Sum2/1 -> zeta/1
  Subsystem/1(zeta(x,t)) -> Sum2/2
  t/1 -> Subsystem1/1(t), Subsystem/1(t)
  x/1 -> Subsystem1/2(x), Subsystem/2(x)

== system Simulator_3D/Subsystem3/Subsystem5 ==
  t : Inport
  x : Inport  Port=2
  Subsystem : Subsystem
  Subsystem1 : Subsystem
  Sum1 : Sum  Inputs=++|
  Sum2 : Sum  Inputs=++|
  zeta : Outport
  theta : Outport  Port=2
  wires:
  x/1 -> Subsystem/2(x), Subsystem1/2(x)
  t/1 -> Subsystem/1(t), Subsystem1/1(t)
  Subsystem/1(zeta(x,t)) -> Sum2/2
  Sum2/1 -> zeta/1
  Subsystem1/1(zeta(x,t)) -> Sum2/1
  Subsystem/2(theta) -> Sum1/2
  Subsystem1/2(theta) -> Sum1/1
  Sum1/1 -> theta/1

== system Simulator_3D/Subsystem3/Subsystem6 ==
  t : Inport
  x : Inport  Port=2
  Subsystem : Subsystem
  Subsystem1 : Subsystem
  Sum1 : Sum  Inputs=++|
  Sum2 : Sum  Inputs=++|
  zeta : Outport
  theta : Outport  Port=2
  wires:
  Sum1/1 -> theta/1
  Subsystem1/2(theta) -> Sum1/1
  Subsystem/2(theta) -> Sum1/2
  Subsystem1/1(zeta(x,t)) -> Sum2/1
  Sum2/1 -> zeta/1
  Subsystem/1(zeta(x,t)) -> Sum2/2
  t/1 -> Subsystem1/1(t), Subsystem/1(t)
  x/1 -> Subsystem1/2(x), Subsystem/2(x)

== system Simulator_3D/Subsystem3/Subsystem7 ==
  t : Inport
  x : Inport  Port=2
  Subsystem : Subsystem
  Subsystem1 : Subsystem
  Sum1 : Sum  Inputs=++|
  Sum2 : Sum  Inputs=++|
  zeta : Outport
  theta : Outport  Port=2
  wires:
  x/1 -> Subsystem/2(x), Subsystem1/2(x)
  t/1 -> Subsystem/1(t), Subsystem1/1(t)
  Subsystem/1(zeta(x,t)) -> Sum2/2
  Sum2/1 -> zeta/1
  Subsystem1/1(zeta(x,t)) -> Sum2/1
  Subsystem/2(theta) -> Sum1/2
  Subsystem1/2(theta) -> Sum1/1
  Sum1/1 -> theta/1

== system Simulator_3D/Subsystem3/Subsystem8 ==
  t : Inport
  x : Inport  Port=2
  Subsystem : Subsystem
  Subsystem1 : Subsystem
  Sum1 : Sum  Inputs=++|
  Sum2 : Sum  Inputs=++|
  zeta : Outport
  theta : Outport  Port=2
  wires:
  Sum1/1 -> theta/1
  Subsystem1/2(theta) -> Sum1/1
  Subsystem/2(theta) -> Sum1/2
  Subsystem1/1(zeta(x,t)) -> Sum2/1
  Sum2/1 -> zeta/1
  Subsystem/1(zeta(x,t)) -> Sum2/2
  t/1 -> Subsystem1/1(t), Subsystem/1(t)
  x/1 -> Subsystem1/2(x), Subsystem/2(x)

== system Simulator_3D/Subsystem3/Subsystem9 ==
  t : Inport
  x : Inport  Port=2
  Subsystem : Subsystem
  Subsystem1 : Subsystem
  Sum1 : Sum  Inputs=++|
  Sum2 : Sum  Inputs=++|
  zeta : Outport
  theta : Outport  Port=2
  wires:
  x/1 -> Subsystem/2(x), Subsystem1/2(x)
  t/1 -> Subsystem/1(t), Subsystem1/1(t)
  Subsystem/1(zeta(x,t)) -> Sum2/2
  Sum2/1 -> zeta/1
  Subsystem1/1(zeta(x,t)) -> Sum2/1
  Subsystem/2(theta) -> Sum1/2
  Subsystem1/2(theta) -> Sum1/1
  Sum1/1 -> theta/1

== system Simulator_3D/Subsystem/5 static wave points/Subsystem12 ==
  t : Inport
  x : Inport  Port=2
  Subsystem : Subsystem
  Subsystem1 : Subsystem
  Sum1 : Sum  Inputs=++|
  Sum2 : Sum  Inputs=++|
  zeta : Outport
  theta : Outport  Port=2
  wires:
  Sum1/1 -> theta/1
  Subsystem1/2(theta) -> Sum1/1
  Subsystem/2(theta) -> Sum1/2
  Subsystem1/1(zeta(x,t)) -> Sum2/1
  Sum2/1 -> zeta/1
  Subsystem/1(zeta(x,t)) -> Sum2/2
  t/1 -> Subsystem1/1(t), Subsystem/1(t)
  x/1 -> Subsystem1/2(x), Subsystem/2(x)

== system Simulator_3D/Subsystem/5 static wave points/Subsystem13 ==
  t : Inport
  x : Inport  Port=2
  Subsystem : Subsystem
  Subsystem1 : Subsystem
  Sum1 : Sum  Inputs=++|
  Sum2 : Sum  Inputs=++|
  zeta : Outport
  theta : Outport  Port=2
  wires:
  x/1 -> Subsystem/2(x), Subsystem1/2(x)
  t/1 -> Subsystem/1(t), Subsystem1/1(t)
  Subsystem/1(zeta(x,t)) -> Sum2/2
  Sum2/1 -> zeta/1
  Subsystem1/1(zeta(x,t)) -> Sum2/1
  Subsystem/2(theta) -> Sum1/2
  Subsystem1/2(theta) -> Sum1/1
  Sum1/1 -> theta/1

== system Simulator_3D/Subsystem/5 static wave points/Subsystem14 ==
  t : Inport
  x : Inport  Port=2
  Subsystem : Subsystem
  Subsystem1 : Subsystem
  Sum1 : Sum  Inputs=++|
  Sum2 : Sum  Inputs=++|
  zeta : Outport
  theta : Outport  Port=2
  wires:
  Sum1/1 -> theta/1
  Subsystem1/2(theta) -> Sum1/1
  Subsystem/2(theta) -> Sum1/2
  Subsystem1/1(zeta(x,t)) -> Sum2/1
  Sum2/1 -> zeta/1
  Subsystem/1(zeta(x,t)) -> Sum2/2
  t/1 -> Subsystem1/1(t), Subsystem/1(t)
  x/1 -> Subsystem1/2(x), Subsystem/2(x)

== system Simulator_3D/Subsystem/5 static wave points/Subsystem15 ==
  t : Inport
  x : Inport  Port=2
  Subsystem : Subsystem
  Subsystem1 : Subsystem
  Sum1 : Sum  Inputs=++|
  Sum2 : Sum  Inputs=++|
  zeta : Outport
  theta : Outport  Port=2
  wires:
  x/1 -> Subsystem/2(x), Subsystem1/2(x)
  t/1 -> Subsystem/1(t), Subsystem1/1(t)
  Subsystem/1(zeta(x,t)) -> Sum2/2
  Sum2/1 -> zeta/1
  Subsystem1/1(zeta(x,t)) -> Sum2/1
  Subsystem/2(theta) -> Sum1/2
  Subsystem1/2(theta) -> Sum1/1
  Sum1/1 -> theta/1

== system Simulator_3D/Subsystem/5 static wave points/Subsystem16 ==
  t : Inport
  x : Inport  Port=2
  Subsystem : Subsystem
  Subsystem1 : Subsystem
  Sum1 : Sum  Inputs=++|
  Sum2 : Sum  Inputs=++|
  zeta : Outport
  theta : Outport  Port=2
  wires:
  Sum1/1 -> theta/1
  Subsystem1/2(theta) -> Sum1/1
  Subsystem/2(theta) -> Sum1/2
  Subsystem1/1(zeta(x,t)) -> Sum2/1
  Sum2/1 -> zeta/1
  Subsystem/1(zeta(x,t)) -> Sum2/2
  t/1 -> Subsystem1/1(t), Subsystem/1(t)
  x/1 -> Subsystem1/2(x), Subsystem/2(x)

== system Simulator_3D/Subsystem/5 static wave points1/Subsystem12 ==
  t : Inport
  x : Inport  Port=2
  Subsystem : Subsystem
  Subsystem1 : Subsystem
  Sum1 : Sum  Inputs=++|
  Sum2 : Sum  Inputs=++|
  zeta : Outport
  theta : Outport  Port=2
  wires:
  Sum1/1 -> theta/1
  Subsystem1/2(theta) -> Sum1/1
  Subsystem/2(theta) -> Sum1/2
  Subsystem1/1(zeta(x,t)) -> Sum2/1
  Sum2/1 -> zeta/1
  Subsystem/1(zeta(x,t)) -> Sum2/2
  t/1 -> Subsystem1/1(t), Subsystem/1(t)
  x/1 -> Subsystem1/2(x), Subsystem/2(x)

== system Simulator_3D/Subsystem/5 static wave points1/Subsystem13 ==
  t : Inport
  x : Inport  Port=2
  Subsystem : Subsystem
  Subsystem1 : Subsystem
  Sum1 : Sum  Inputs=++|
  Sum2 : Sum  Inputs=++|
  zeta : Outport
  theta : Outport  Port=2
  wires:
  x/1 -> Subsystem/2(x), Subsystem1/2(x)
  t/1 -> Subsystem/1(t), Subsystem1/1(t)
  Subsystem/1(zeta(x,t)) -> Sum2/2
  Sum2/1 -> zeta/1
  Subsystem1/1(zeta(x,t)) -> Sum2/1
  Subsystem/2(theta) -> Sum1/2
  Subsystem1/2(theta) -> Sum1/1
  Sum1/1 -> theta/1

== system Simulator_3D/Subsystem/5 static wave points1/Subsystem14 ==
  t : Inport
  x : Inport  Port=2
  Subsystem : Subsystem
  Subsystem1 : Subsystem
  Sum1 : Sum  Inputs=++|
  Sum2 : Sum  Inputs=++|
  zeta : Outport
  theta : Outport  Port=2
  wires:
  Sum1/1 -> theta/1
  Subsystem1/2(theta) -> Sum1/1
  Subsystem/2(theta) -> Sum1/2
  Subsystem1/1(zeta(x,t)) -> Sum2/1
  Sum2/1 -> zeta/1
  Subsystem/1(zeta(x,t)) -> Sum2/2
  t/1 -> Subsystem1/1(t), Subsystem/1(t)
  x/1 -> Subsystem1/2(x), Subsystem/2(x)

== system Simulator_3D/Subsystem/5 static wave points1/Subsystem15 ==
  t : Inport
  x : Inport  Port=2
  Subsystem : Subsystem
  Subsystem1 : Subsystem
  Sum1 : Sum  Inputs=++|
  Sum2 : Sum  Inputs=++|
  zeta : Outport
  theta : Outport  Port=2
  wires:
  x/1 -> Subsystem/2(x), Subsystem1/2(x)
  t/1 -> Subsystem/1(t), Subsystem1/1(t)
  Subsystem/1(zeta(x,t)) -> Sum2/2
  Sum2/1 -> zeta/1
  Subsystem1/1(zeta(x,t)) -> Sum2/1
  Subsystem/2(theta) -> Sum1/2
  Subsystem1/2(theta) -> Sum1/1
  Sum1/1 -> theta/1

== system Simulator_3D/Subsystem/5 static wave points1/Subsystem16 ==
  t : Inport
  x : Inport  Port=2
  Subsystem : Subsystem
  Subsystem1 : Subsystem
  Sum1 : Sum  Inputs=++|
  Sum2 : Sum  Inputs=++|
  zeta : Outport
  theta : Outport  Port=2
  wires:
  Sum1/1 -> theta/1
  Subsystem1/2(theta) -> Sum1/1
  Subsystem/2(theta) -> Sum1/2
  Subsystem1/1(zeta(x,t)) -> Sum2/1
  Sum2/1 -> zeta/1
  Subsystem/1(zeta(x,t)) -> Sum2/2
  t/1 -> Subsystem1/1(t), Subsystem/1(t)
  x/1 -> Subsystem1/2(x), Subsystem/2(x)

== system Simulator_3D/Subsystem/5 static wave points2/Subsystem12 ==
  t : Inport
  x : Inport  Port=2
  Subsystem : Subsystem
  Subsystem1 : Subsystem
  Sum1 : Sum  Inputs=++|
  Sum2 : Sum  Inputs=++|
  zeta : Outport
  theta : Outport  Port=2
  wires:
  Sum1/1 -> theta/1
  Subsystem1/2(theta) -> Sum1/1
  Subsystem/2(theta) -> Sum1/2
  Subsystem1/1(zeta(x,t)) -> Sum2/1
  Sum2/1 -> zeta/1
  Subsystem/1(zeta(x,t)) -> Sum2/2
  t/1 -> Subsystem1/1(t), Subsystem/1(t)
  x/1 -> Subsystem1/2(x), Subsystem/2(x)

== system Simulator_3D/Subsystem/5 static wave points2/Subsystem13 ==
  t : Inport
  x : Inport  Port=2
  Subsystem : Subsystem
  Subsystem1 : Subsystem
  Sum1 : Sum  Inputs=++|
  Sum2 : Sum  Inputs=++|
  zeta : Outport
  theta : Outport  Port=2
  wires:
  x/1 -> Subsystem/2(x), Subsystem1/2(x)
  t/1 -> Subsystem/1(t), Subsystem1/1(t)
  Subsystem/1(zeta(x,t)) -> Sum2/2
  Sum2/1 -> zeta/1
  Subsystem1/1(zeta(x,t)) -> Sum2/1
  Subsystem/2(theta) -> Sum1/2
  Subsystem1/2(theta) -> Sum1/1
  Sum1/1 -> theta/1

== system Simulator_3D/Subsystem/5 static wave points2/Subsystem14 ==
  t : Inport
  x : Inport  Port=2
  Subsystem : Subsystem
  Subsystem1 : Subsystem
  Sum1 : Sum  Inputs=++|
  Sum2 : Sum  Inputs=++|
  zeta : Outport
  theta : Outport  Port=2
  wires:
  Sum1/1 -> theta/1
  Subsystem1/2(theta) -> Sum1/1
  Subsystem/2(theta) -> Sum1/2
  Subsystem1/1(zeta(x,t)) -> Sum2/1
  Sum2/1 -> zeta/1
  Subsystem/1(zeta(x,t)) -> Sum2/2
  t/1 -> Subsystem1/1(t), Subsystem/1(t)
  x/1 -> Subsystem1/2(x), Subsystem/2(x)

== system Simulator_3D/Subsystem/5 static wave points2/Subsystem15 ==
  t : Inport
  x : Inport  Port=2
  Subsystem : Subsystem
  Subsystem1 : Subsystem
  Sum1 : Sum  Inputs=++|
  Sum2 : Sum  Inputs=++|
  zeta : Outport
  theta : Outport  Port=2
  wires:
  x/1 -> Subsystem/2(x), Subsystem1/2(x)
  t/1 -> Subsystem/1(t), Subsystem1/1(t)
  Subsystem/1(zeta(x,t)) -> Sum2/2
  Sum2/1 -> zeta/1
  Subsystem1/1(zeta(x,t)) -> Sum2/1
  Subsystem/2(theta) -> Sum1/2
  Subsystem1/2(theta) -> Sum1/1
  Sum1/1 -> theta/1

== system Simulator_3D/Subsystem/5 static wave points2/Subsystem16 ==
  t : Inport
  x : Inport  Port=2
  Subsystem : Subsystem
  Subsystem1 : Subsystem
  Sum1 : Sum  Inputs=++|
  Sum2 : Sum  Inputs=++|
  zeta : Outport
  theta : Outport  Port=2
  wires:
  Sum1/1 -> theta/1
  Subsystem1/2(theta) -> Sum1/1
  Subsystem/2(theta) -> Sum1/2
  Subsystem1/1(zeta(x,t)) -> Sum2/1
  Sum2/1 -> zeta/1
  Subsystem/1(zeta(x,t)) -> Sum2/2
  t/1 -> Subsystem1/1(t), Subsystem/1(t)
  x/1 -> Subsystem1/2(x), Subsystem/2(x)

== system Simulator_3D/Subsystem/5 static wave points3/Subsystem1 ==
  t : Inport
  x : Inport  Port=2
  Subsystem : Subsystem
  Subsystem1 : Subsystem
  Sum1 : Sum  Inputs=++|
  Sum2 : Sum  Inputs=++|
  zeta : Outport
  theta : Outport  Port=2
  wires:
  x/1 -> Subsystem/2(x), Subsystem1/2(x)
  t/1 -> Subsystem/1(t), Subsystem1/1(t)
  Subsystem/1(zeta(x,t)) -> Sum2/2
  Sum2/1 -> zeta/1
  Subsystem1/1(zeta(x,t)) -> Sum2/1
  Subsystem/2(theta) -> Sum1/2
  Subsystem1/2(theta) -> Sum1/1
  Sum1/1 -> theta/1

== system Simulator_3D/Subsystem/5 static wave points3/Subsystem12 ==
  t : Inport
  x : Inport  Port=2
  Subsystem : Subsystem
  Subsystem1 : Subsystem
  Sum1 : Sum  Inputs=++|
  Sum2 : Sum  Inputs=++|
  zeta : Outport
  theta : Outport  Port=2
  wires:
  Sum1/1 -> theta/1
  Subsystem1/2(theta) -> Sum1/1
  Subsystem/2(theta) -> Sum1/2
  Subsystem1/1(zeta(x,t)) -> Sum2/1
  Sum2/1 -> zeta/1
  Subsystem/1(zeta(x,t)) -> Sum2/2
  t/1 -> Subsystem1/1(t), Subsystem/1(t)
  x/1 -> Subsystem1/2(x), Subsystem/2(x)

== system Simulator_3D/Subsystem/5 static wave points3/Subsystem13 ==
  t : Inport
  x : Inport  Port=2
  Subsystem : Subsystem
  Subsystem1 : Subsystem
  Sum1 : Sum  Inputs=++|
  Sum2 : Sum  Inputs=++|
  zeta : Outport
  theta : Outport  Port=2
  wires:
  x/1 -> Subsystem/2(x), Subsystem1/2(x)
  t/1 -> Subsystem/1(t), Subsystem1/1(t)
  Subsystem/1(zeta(x,t)) -> Sum2/2
  Sum2/1 -> zeta/1
  Subsystem1/1(zeta(x,t)) -> Sum2/1
  Subsystem/2(theta) -> Sum1/2
  Subsystem1/2(theta) -> Sum1/1
  Sum1/1 -> theta/1

== system Simulator_3D/Subsystem/5 static wave points3/Subsystem14 ==
  t : Inport
  x : Inport  Port=2
  Subsystem : Subsystem
  Subsystem1 : Subsystem
  Sum1 : Sum  Inputs=++|
  Sum2 : Sum  Inputs=++|
  zeta : Outport
  theta : Outport  Port=2
  wires:
  Sum1/1 -> theta/1
  Subsystem1/2(theta) -> Sum1/1
  Subsystem/2(theta) -> Sum1/2
  Subsystem1/1(zeta(x,t)) -> Sum2/1
  Sum2/1 -> zeta/1
  Subsystem/1(zeta(x,t)) -> Sum2/2
  t/1 -> Subsystem1/1(t), Subsystem/1(t)
  x/1 -> Subsystem1/2(x), Subsystem/2(x)

== system Simulator_3D/Subsystem/5 static wave points3/Subsystem15 ==
  t : Inport
  x : Inport  Port=2
  Subsystem : Subsystem
  Subsystem1 : Subsystem
  Sum1 : Sum  Inputs=++|
  Sum2 : Sum  Inputs=++|
  zeta : Outport
  theta : Outport  Port=2
  wires:
  x/1 -> Subsystem/2(x), Subsystem1/2(x)
  t/1 -> Subsystem/1(t), Subsystem1/1(t)
  Subsystem/1(zeta(x,t)) -> Sum2/2
  Sum2/1 -> zeta/1
  Subsystem1/1(zeta(x,t)) -> Sum2/1
  Subsystem/2(theta) -> Sum1/2
  Subsystem1/2(theta) -> Sum1/1
  Sum1/1 -> theta/1

== system Simulator_3D/Subsystem/5 static wave points3/Subsystem16 ==
  t : Inport
  x : Inport  Port=2
  Subsystem : Subsystem
  Subsystem1 : Subsystem
  Sum1 : Sum  Inputs=++|
  Sum2 : Sum  Inputs=++|
  zeta : Outport
  theta : Outport  Port=2
  wires:
  Sum1/1 -> theta/1
  Subsystem1/2(theta) -> Sum1/1
  Subsystem/2(theta) -> Sum1/2
  Subsystem1/1(zeta(x,t)) -> Sum2/1
  Sum2/1 -> zeta/1
  Subsystem/1(zeta(x,t)) -> Sum2/2
  t/1 -> Subsystem1/1(t), Subsystem/1(t)
  x/1 -> Subsystem1/2(x), Subsystem/2(x)

== system Simulator_3D/Subsystem/5 static wave points3/Subsystem2 ==
  t : Inport
  x : Inport  Port=2
  Subsystem : Subsystem
  Subsystem1 : Subsystem
  Sum1 : Sum  Inputs=++|
  Sum2 : Sum  Inputs=++|
  zeta : Outport
  theta : Outport  Port=2
  wires:
  Sum1/1 -> theta/1
  Subsystem1/2(theta) -> Sum1/1
  Subsystem/2(theta) -> Sum1/2
  Subsystem1/1(zeta(x,t)) -> Sum2/1
  Sum2/1 -> zeta/1
  Subsystem/1(zeta(x,t)) -> Sum2/2
  t/1 -> Subsystem1/1(t), Subsystem/1(t)
  x/1 -> Subsystem1/2(x), Subsystem/2(x)

== system Simulator_3D/Subsystem/5 static wave points3/Subsystem3 ==
  t : Inport
  x : Inport  Port=2
  Subsystem : Subsystem
  Subsystem1 : Subsystem
  Sum1 : Sum  Inputs=++|
  Sum2 : Sum  Inputs=++|
  zeta : Outport
  theta : Outport  Port=2
  wires:
  x/1 -> Subsystem/2(x), Subsystem1/2(x)
  t/1 -> Subsystem/1(t), Subsystem1/1(t)
  Subsystem/1(zeta(x,t)) -> Sum2/2
  Sum2/1 -> zeta/1
  Subsystem1/1(zeta(x,t)) -> Sum2/1
  Subsystem/2(theta) -> Sum1/2
  Subsystem1/2(theta) -> Sum1/1
  Sum1/1 -> theta/1

== system Simulator_3D/Subsystem/5 static wave points4/Subsystem12 ==
  t : Inport
  x : Inport  Port=2
  Subsystem : Subsystem
  Subsystem1 : Subsystem
  Sum1 : Sum  Inputs=++|
  Sum2 : Sum  Inputs=++|
  zeta : Outport
  theta : Outport  Port=2
  wires:
  x/1 -> Subsystem/2(x), Subsystem1/2(x)
  t/1 -> Subsystem/1(t), Subsystem1/1(t)
  Subsystem/1(zeta(x,t)) -> Sum2/2
  Sum2/1 -> zeta/1
  Subsystem1/1(zeta(x,t)) -> Sum2/1
  Subsystem/2(theta) -> Sum1/2
  Subsystem1/2(theta) -> Sum1/1
  Sum1/1 -> theta/1

== system Simulator_3D/Subsystem/5 static wave points4/Subsystem13 ==
  t : Inport
  x : Inport  Port=2
  Subsystem : Subsystem
  Subsystem1 : Subsystem
  Sum1 : Sum  Inputs=++|
  Sum2 : Sum  Inputs=++|
  zeta : Outport
  theta : Outport  Port=2
  wires:
  Sum1/1 -> theta/1
  Subsystem1/2(theta) -> Sum1/1
  Subsystem/2(theta) -> Sum1/2
  Subsystem1/1(zeta(x,t)) -> Sum2/1
  Sum2/1 -> zeta/1
  Subsystem/1(zeta(x,t)) -> Sum2/2
  t/1 -> Subsystem1/1(t), Subsystem/1(t)
  x/1 -> Subsystem1/2(x), Subsystem/2(x)

== system Simulator_3D/Subsystem/5 static wave points4/Subsystem14 ==
  t : Inport
  x : Inport  Port=2
  Subsystem : Subsystem
  Subsystem1 : Subsystem
  Sum1 : Sum  Inputs=++|
  Sum2 : Sum  Inputs=++|
  zeta : Outport
  theta : Outport  Port=2
  wires:
  x/1 -> Subsystem/2(x), Subsystem1/2(x)
  t/1 -> Subsystem/1(t), Subsystem1/1(t)
  Subsystem/1(zeta(x,t)) -> Sum2/2
  Sum2/1 -> zeta/1
  Subsystem1/1(zeta(x,t)) -> Sum2/1
  Subsystem/2(theta) -> Sum1/2
  Subsystem1/2(theta) -> Sum1/1
  Sum1/1 -> theta/1

== system Simulator_3D/Subsystem/5 static wave points4/Subsystem15 ==
  t : Inport
  x : Inport  Port=2
  Subsystem : Subsystem
  Subsystem1 : Subsystem
  Sum1 : Sum  Inputs=++|
  Sum2 : Sum  Inputs=++|
  zeta : Outport
  theta : Outport  Port=2
  wires:
  Sum1/1 -> theta/1
  Subsystem1/2(theta) -> Sum1/1
  Subsystem/2(theta) -> Sum1/2
  Subsystem1/1(zeta(x,t)) -> Sum2/1
  Sum2/1 -> zeta/1
  Subsystem/1(zeta(x,t)) -> Sum2/2
  t/1 -> Subsystem1/1(t), Subsystem/1(t)
  x/1 -> Subsystem1/2(x), Subsystem/2(x)

== system Simulator_3D/Subsystem/5 static wave points4/Subsystem16 ==
  t : Inport
  x : Inport  Port=2
  Subsystem : Subsystem
  Subsystem1 : Subsystem
  Sum1 : Sum  Inputs=++|
  Sum2 : Sum  Inputs=++|
  zeta : Outport
  theta : Outport  Port=2
  wires:
  x/1 -> Subsystem/2(x), Subsystem1/2(x)
  t/1 -> Subsystem/1(t), Subsystem1/1(t)
  Subsystem/1(zeta(x,t)) -> Sum2/2
  Sum2/1 -> zeta/1
  Subsystem1/1(zeta(x,t)) -> Sum2/1
  Subsystem/2(theta) -> Sum1/2
  Subsystem1/2(theta) -> Sum1/1
  Sum1/1 -> theta/1

== system Simulator_3D/Subsystem/5 static wave points5/Subsystem12 ==
  t : Inport
  x : Inport  Port=2
  Subsystem : Subsystem
  Subsystem1 : Subsystem
  Sum1 : Sum  Inputs=++|
  Sum2 : Sum  Inputs=++|
  zeta : Outport
  theta : Outport  Port=2
  wires:
  Sum1/1 -> theta/1
  Subsystem1/2(theta) -> Sum1/1
  Subsystem/2(theta) -> Sum1/2
  Subsystem1/1(zeta(x,t)) -> Sum2/1
  Sum2/1 -> zeta/1
  Subsystem/1(zeta(x,t)) -> Sum2/2
  t/1 -> Subsystem1/1(t), Subsystem/1(t)
  x/1 -> Subsystem1/2(x), Subsystem/2(x)

== system Simulator_3D/Subsystem/5 static wave points5/Subsystem13 ==
  t : Inport
  x : Inport  Port=2
  Subsystem : Subsystem
  Subsystem1 : Subsystem
  Sum1 : Sum  Inputs=++|
  Sum2 : Sum  Inputs=++|
  zeta : Outport
  theta : Outport  Port=2
  wires:
  x/1 -> Subsystem/2(x), Subsystem1/2(x)
  t/1 -> Subsystem/1(t), Subsystem1/1(t)
  Subsystem/1(zeta(x,t)) -> Sum2/2
  Sum2/1 -> zeta/1
  Subsystem1/1(zeta(x,t)) -> Sum2/1
  Subsystem/2(theta) -> Sum1/2
  Subsystem1/2(theta) -> Sum1/1
  Sum1/1 -> theta/1

== system Simulator_3D/Subsystem/5 static wave points5/Subsystem14 ==
  t : Inport
  x : Inport  Port=2
  Subsystem : Subsystem
  Subsystem1 : Subsystem
  Sum1 : Sum  Inputs=++|
  Sum2 : Sum  Inputs=++|
  zeta : Outport
  theta : Outport  Port=2
  wires:
  Sum1/1 -> theta/1
  Subsystem1/2(theta) -> Sum1/1
  Subsystem/2(theta) -> Sum1/2
  Subsystem1/1(zeta(x,t)) -> Sum2/1
  Sum2/1 -> zeta/1
  Subsystem/1(zeta(x,t)) -> Sum2/2
  t/1 -> Subsystem1/1(t), Subsystem/1(t)
  x/1 -> Subsystem1/2(x), Subsystem/2(x)

== system Simulator_3D/Subsystem/5 static wave points5/Subsystem15 ==
  t : Inport
  x : Inport  Port=2
  Subsystem : Subsystem
  Subsystem1 : Subsystem
  Sum1 : Sum  Inputs=++|
  Sum2 : Sum  Inputs=++|
  zeta : Outport
  theta : Outport  Port=2
  wires:
  x/1 -> Subsystem/2(x), Subsystem1/2(x)
  t/1 -> Subsystem/1(t), Subsystem1/1(t)
  Subsystem/1(zeta(x,t)) -> Sum2/2
  Sum2/1 -> zeta/1
  Subsystem1/1(zeta(x,t)) -> Sum2/1
  Subsystem/2(theta) -> Sum1/2
  Subsystem1/2(theta) -> Sum1/1
  Sum1/1 -> theta/1

== system Simulator_3D/Subsystem/5 static wave points5/Subsystem16 ==
  t : Inport
  x : Inport  Port=2
  Subsystem : Subsystem
  Subsystem1 : Subsystem
  Sum1 : Sum  Inputs=++|
  Sum2 : Sum  Inputs=++|
  zeta : Outport
  theta : Outport  Port=2
  wires:
  Sum1/1 -> theta/1
  Subsystem1/2(theta) -> Sum1/1
  Subsystem/2(theta) -> Sum1/2
  Subsystem1/1(zeta(x,t)) -> Sum2/1
  Sum2/1 -> zeta/1
  Subsystem/1(zeta(x,t)) -> Sum2/2
  t/1 -> Subsystem1/1(t), Subsystem/1(t)
  x/1 -> Subsystem1/2(x), Subsystem/2(x)

== system Simulator_3D/Subsystem/5 static wave points6/Subsystem12 ==
  t : Inport
  x : Inport  Port=2
  Subsystem : Subsystem
  Subsystem1 : Subsystem
  Sum1 : Sum  Inputs=++|
  Sum2 : Sum  Inputs=++|
  zeta : Outport
  theta : Outport  Port=2
  wires:
  x/1 -> Subsystem/2(x), Subsystem1/2(x)
  t/1 -> Subsystem/1(t), Subsystem1/1(t)
  Subsystem/1(zeta(x,t)) -> Sum2/2
  Sum2/1 -> zeta/1
  Subsystem1/1(zeta(x,t)) -> Sum2/1
  Subsystem/2(theta) -> Sum1/2
  Subsystem1/2(theta) -> Sum1/1
  Sum1/1 -> theta/1

== system Simulator_3D/Subsystem/5 static wave points6/Subsystem13 ==
  t : Inport
  x : Inport  Port=2
  Subsystem : Subsystem
  Subsystem1 : Subsystem
  Sum1 : Sum  Inputs=++|
  Sum2 : Sum  Inputs=++|
  zeta : Outport
  theta : Outport  Port=2
  wires:
  Sum1/1 -> theta/1
  Subsystem1/2(theta) -> Sum1/1
  Subsystem/2(theta) -> Sum1/2
  Subsystem1/1(zeta(x,t)) -> Sum2/1
  Sum2/1 -> zeta/1
  Subsystem/1(zeta(x,t)) -> Sum2/2
  t/1 -> Subsystem1/1(t), Subsystem/1(t)
  x/1 -> Subsystem1/2(x), Subsystem/2(x)

== system Simulator_3D/Subsystem/5 static wave points6/Subsystem14 ==
  t : Inport
  x : Inport  Port=2
  Subsystem : Subsystem
  Subsystem1 : Subsystem
  Sum1 : Sum  Inputs=++|
  Sum2 : Sum  Inputs=++|
  zeta : Outport
  theta : Outport  Port=2
  wires:
  x/1 -> Subsystem/2(x), Subsystem1/2(x)
  t/1 -> Subsystem/1(t), Subsystem1/1(t)
  Subsystem/1(zeta(x,t)) -> Sum2/2
  Sum2/1 -> zeta/1
  Subsystem1/1(zeta(x,t)) -> Sum2/1
  Subsystem/2(theta) -> Sum1/2
  Subsystem1/2(theta) -> Sum1/1
  Sum1/1 -> theta/1

== system Simulator_3D/Subsystem/5 static wave points6/Subsystem15 ==
  t : Inport
  x : Inport  Port=2
  Subsystem : Subsystem
  Subsystem1 : Subsystem
  Sum1 : Sum  Inputs=++|
  Sum2 : Sum  Inputs=++|
  zeta : Outport
  theta : Outport  Port=2
  wires:
  Sum1/1 -> theta/1
  Subsystem1/2(theta) -> Sum1/1
  Subsystem/2(theta) -> Sum1/2
  Subsystem1/1(zeta(x,t)) -> Sum2/1
  Sum2/1 -> zeta/1
  Subsystem/1(zeta(x,t)) -> Sum2/2
  t/1 -> Subsystem1/1(t), Subsystem/1(t)
  x/1 -> Subsystem1/2(x), Subsystem/2(x)
